simulink model "provaSimulink"  (R2023b)
settings: Solver=VariableStepAuto  StartTime=0.04  StopTime=41.84  RelTol=1e-3
values from neighbouring files (symbols this model uses):
  acc = db.data(inizio:fine,2:4)*mRot*g*1e-3    [laSalvezzaForse.m]    (also in laSperanzaForse.m = lowpass(acc,1,25); loadData.m = db(inizio:fine,2:4)*gRot*9.81/-gMedio; nuovoApproccio.m = lowpass(acc,1,25); nuovoApproccio2.m = lowpass(acc,1,25))
  vang = db.data(inizio:fine,5:7)*2*pi/360*1e-3    [laSalvezzaForse.m]    (also in laSperanzaForse.m = lowpass(vang,1,25); loadData.m = db(inizio:fine,5:7)*gRot*2*pi/360*1e-3; nuovoApproccio.m = lowpass(vang,1,25); nuovoApproccio2.m = lowpass(vang,1,25))
libraries: mspfiltlib x1
settings Model: Creator=Daniele  LastModifiedBy=Daniele
settings DataIOCC: TimeSaveName=t

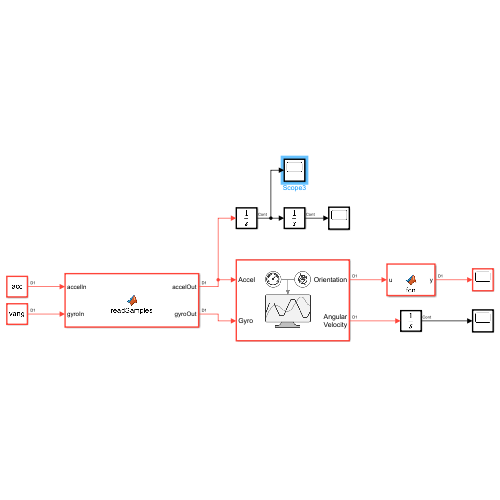
[thumbnail: Simulink's stored preview of the top-level diagram]
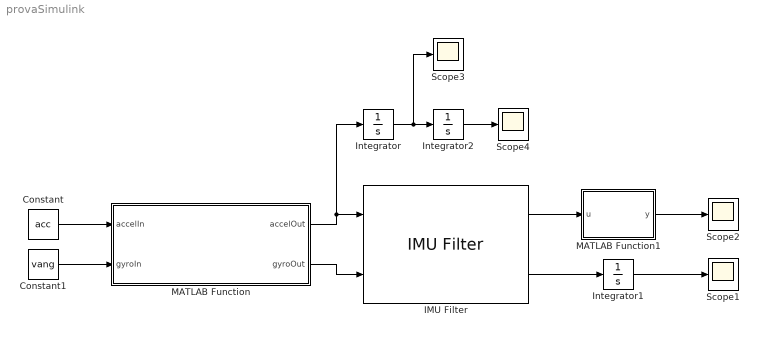
== system provaSimulink ==
  Constant : Constant  Value=acc  SampleTime=0.04
  Constant1 : Constant  Value=vang  SampleTime=0.04
  IMU Filter : mspfiltlib/IMU Filter  DispRefFrame=ENU  OrientationFormat=quaternion  DecimationFactor=1  InitialProcessNoise=imufilter.defaultProcessNoise  AccelerometerNoise=0.0001924722  GyroscopeNoise=9.1385e-5  GyroscopeDriftNoise=3.0462e-13  LinearAccelerationNoise=0.0096236100000000012  LinearAccelerationDecayFactor=0.5  SimulateUsing=Interpreted execution
  Integrator : Integrator
  Integrator1 : Integrator
  Integrator2 : Integrator
  MATLAB Function : MATLAB Function  TreatAsAtomicUnit=on
  MATLAB Function1 : MATLAB Function  TreatAsAtomicUnit=on
  Scope{1..4} (4 alike) : Scope
  wires:
  MATLAB Function/1(accelOut) -> Integrator/1, IMU Filter/1
  MATLAB Function/2(gyroOut) -> IMU Filter/2
  Constant/1 -> MATLAB Function/1(accelIn)
  Constant1/1 -> MATLAB Function/2(gyroIn)
  IMU Filter/1 -> MATLAB Function1/1(u)
  MATLAB Function1/1(y) -> Scope2/1
  IMU Filter/2 -> Integrator1/1
  Integrator/1 -> Integrator2/1, Scope3/1
  Integrator1/1 -> Scope1/1
  Integrator2/1 -> Scope4/1

== matlab function provaSimulink/MATLAB Function ==
  data: accelOut output; gyroOut output; accelIn input; gyroIn input
function [accelOut,gyroOut] = readSamples(accelIn,gyroIn)

persistent selectSample;
if isempty(selectSample)
    selectSample = 0;
end
selectSample = selectSample + 1;

accelOut = accelIn(selectSample,:);
gyroOut = gyroIn(selectSample,:);

== matlab function provaSimulink/MATLAB Function1 ==
  data: u input; y output
function y = fcn(u)

q2 = quaternion(u(:,1), u(:,2), u(:,3), u(:,4));
y=euler(q2,'XYZ','frame');
